simulink model "test"  (R2020b)
settings: Solver=FixedStepAuto  StartTime=0.0  StopTime=10.0  RelTol=1e-3
settings Model: Creator=horse  LastModifiedBy=faith
settings OptimizationCC: BlockReduction=off  ConditionallyExecuteInputs=off  DefaultParameterBehavior=Inlined  OptimizeBlockIOStorage=off
settings HardwareCC: TargetBitPerPointer=64  TargetBitPerSizeT=64  TargetBitPerPtrDiffT=64  TargetLongLongMode=on  TargetIntDivRoundTo=Zero  TargetEndianess=LittleEndian  TargetWordSize=64  TargetHWDeviceType=Generic->Custom  ProdEqTarget=off
settings RTWCC: Description=SystemVerilog DPI Component Generator  SystemTargetFile=systemverilog_dpi_grt.tlc  TemplateMakefile=systemverilog_dpi_grt_default_tmf
settings CodeAppCC: MaxIdLength=256
settings DPIGRTTargetCC: TargetFcnLib=ansi_tfl_table_tmw.mat  GenFloatMathFcnCalls=NOT IN USE  TargetLangStandard=C89/C90 (ANSI)  CodeReplacementLibrary=None  UtilityFuncGeneration=Auto  MultiwordTypeDef=System defined  MultiwordLength=2048  DynamicStringBufferSize=256  GenerateFullHeader=on  InferredTypesCompatibility=off  GenerateSampleERTMain=off  GenerateTestInterfaces=off  ModelReferenceCompliant=on  ParMdlRefBuildCompliant=on  CompOptLevelCompliant=off  ConcurrentExecutionCompliant=off  IncludeMdlTerminateFcn=on  CombineOutputUpdateFcns=off  CombineSignalStateStructs=on  GroupInternalDataByFunction=off  SuppressErrorStatus=off  IncludeFileDelimiter=Auto  ERTCustomFileBanners=off  SupportAbsoluteTime=on  LogVarNameModifier=rt_  MatFileLogging=off  CodeInterfacePackaging=Reusable function  PurelyIntegerCode=off  SupportNonFinite=on  SupportComplex=on  SupportContinuousTime=on  SupportNonInlinedSFcns=on  RemoveDisableFunc=off  RemoveResetFunc=off  SupportVariableSizeSignals=off  ParenthesesLevel=Nominal  CastingMode=Nominal  MATLABClassNameForMDSCustomization=Simulink.SoftwareTarget.TargetSpecificTriggerConfigurationBase  ModelStepFunctionPrototypeControlCompliant=off  CPPClassGenCompliant=off  AutosarCompliant=off  MDXCompliant=off  GRTInterface=off  GenerateAllocFcn=on  UseToolchainInfoCompliant=on  GenerateSharedConstants=on  CoderGroups=[]  AccessMethods=[]  LookupTableObjectStructAxisOrder=1,2,3,4,...  LUTObjectStructOrderExplicitValues=Size,Breakpoints,Table  LUTObjectStructOrderEvenSpacing=Size,Breakpoints,Table  ArrayLayout=Column-major  UnsupportedSFcnMsg=error  ERTHeaderFileRootName=$R$E  ERTSourceFileRootName=$R$E  ERTDataFileRootName=$R_data  RTWCAPISignals=on  RTWCAPIParams=off  RTWCAPIStates=off  RTWCAPIRootIO=off  ExtMode=off  ExtModeTransport=0  ExtModeStaticAlloc=off  ExtModeStaticAllocSize=1000000  ExtModeTesting=off  ExtModeMexFile=ext_comm  GenerateASAP2=off  MultiInstanceErrorCode=Error  DPICustomizeSystemVerilogCode=off  DPISystemVerilogTemplate=svdpi_event.vgt  DPIReportRunTimeError=off  DPIRunTimeErrorSeverity=Fatal  DPIGenerateTestBench=off  DPITestBenchSimulator=Mentor Graphics Questasim  DPITestPointAccessFcnInterface=None  DPIFixedPointDataType=CompatibleCType  DPIPortConnection=Port list  DPICompositeDataType=Flattened

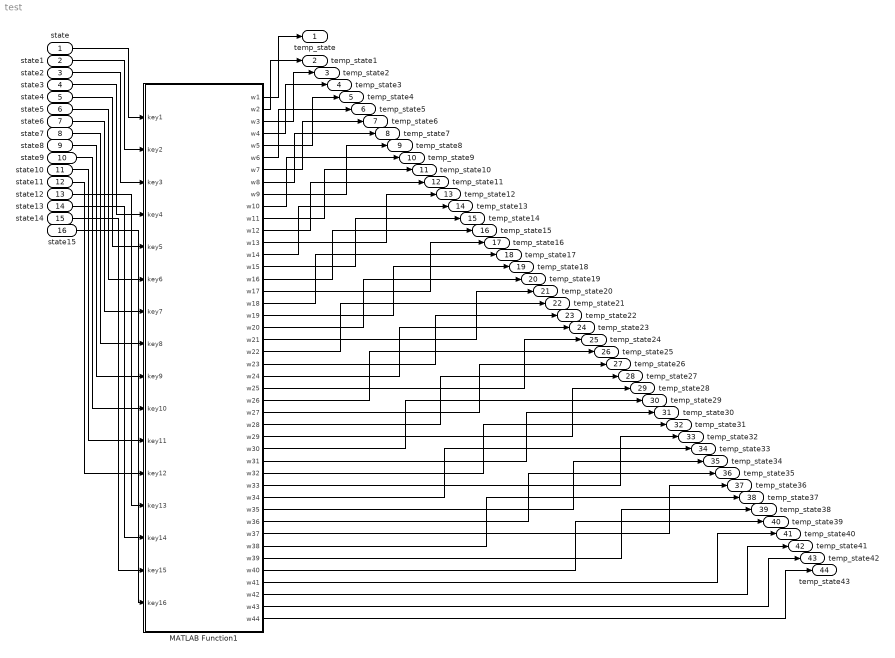
== system test ==
  state : Inport  OutDataTypeStr=uint8
  state1 : Inport  Port=2  OutDataTypeStr=uint8
  state2 : Inport  Port=3  OutDataTypeStr=uint8
  state3 : Inport  Port=4  OutDataTypeStr=uint8
  state4 : Inport  Port=5  OutDataTypeStr=uint8
  state5 : Inport  Port=6  OutDataTypeStr=uint8
  state6 : Inport  Port=7  OutDataTypeStr=uint8
  state7 : Inport  Port=8  OutDataTypeStr=uint8
  state8 : Inport  Port=9  OutDataTypeStr=uint8
  state9 : Inport  Port=10  OutDataTypeStr=uint8
  state10 : Inport  Port=11  OutDataTypeStr=uint8
  state11 : Inport  Port=12  OutDataTypeStr=uint8
  state12 : Inport  Port=13  OutDataTypeStr=uint8
  state13 : Inport  Port=14  OutDataTypeStr=uint8
  state14 : Inport  Port=15  OutDataTypeStr=uint8
  state15 : Inport  Port=16  OutDataTypeStr=uint8
  MATLAB Function1 : MATLAB Function  TreatAsAtomicUnit=on
  temp_state : Outport  OutDataTypeStr=uint32  VectorParamsAs1DForOutWhenUnconnected=off
  temp_state1 : Outport  Port=2  OutDataTypeStr=uint32  VectorParamsAs1DForOutWhenUnconnected=off
  temp_state2 : Outport  Port=3  OutDataTypeStr=uint32  VectorParamsAs1DForOutWhenUnconnected=off
  temp_state3 : Outport  Port=4  OutDataTypeStr=uint32  VectorParamsAs1DForOutWhenUnconnected=off
  temp_state4 : Outport  Port=5  OutDataTypeStr=uint32  VectorParamsAs1DForOutWhenUnconnected=off
  temp_state5 : Outport  Port=6  OutDataTypeStr=uint32  VectorParamsAs1DForOutWhenUnconnected=off
  temp_state6 : Outport  Port=7  OutDataTypeStr=uint32  VectorParamsAs1DForOutWhenUnconnected=off
  temp_state7 : Outport  Port=8  OutDataTypeStr=uint32  VectorParamsAs1DForOutWhenUnconnected=off
  temp_state8 : Outport  Port=9  OutDataTypeStr=uint32  VectorParamsAs1DForOutWhenUnconnected=off
  temp_state9 : Outport  Port=10  OutDataTypeStr=uint32  VectorParamsAs1DForOutWhenUnconnected=off
  temp_state10 : Outport  Port=11  OutDataTypeStr=uint32  VectorParamsAs1DForOutWhenUnconnected=off
  temp_state11 : Outport  Port=12  OutDataTypeStr=uint32  VectorParamsAs1DForOutWhenUnconnected=off
  temp_state12 : Outport  Port=13  OutDataTypeStr=uint32  VectorParamsAs1DForOutWhenUnconnected=off
  temp_state13 : Outport  Port=14  OutDataTypeStr=uint32  VectorParamsAs1DForOutWhenUnconnected=off
  temp_state14 : Outport  Port=15  OutDataTypeStr=uint32  VectorParamsAs1DForOutWhenUnconnected=off
  temp_state15 : Outport  Port=16  OutDataTypeStr=uint32  VectorParamsAs1DForOutWhenUnconnected=off
  temp_state16 : Outport  Port=17  OutDataTypeStr=uint32  VectorParamsAs1DForOutWhenUnconnected=off
  temp_state17 : Outport  Port=18  OutDataTypeStr=uint32  VectorParamsAs1DForOutWhenUnconnected=off
  temp_state18 : Outport  Port=19  OutDataTypeStr=uint32  VectorParamsAs1DForOutWhenUnconnected=off
  temp_state19 : Outport  Port=20  OutDataTypeStr=uint32  VectorParamsAs1DForOutWhenUnconnected=off
  temp_state20 : Outport  Port=21  OutDataTypeStr=uint32  VectorParamsAs1DForOutWhenUnconnected=off
  temp_state21 : Outport  Port=22  OutDataTypeStr=uint32  VectorParamsAs1DForOutWhenUnconnected=off
  temp_state22 : Outport  Port=23  OutDataTypeStr=uint32  VectorParamsAs1DForOutWhenUnconnected=off
  temp_state23 : Outport  Port=24  OutDataTypeStr=uint32  VectorParamsAs1DForOutWhenUnconnected=off
  temp_state24 : Outport  Port=25  OutDataTypeStr=uint32  VectorParamsAs1DForOutWhenUnconnected=off
  temp_state25 : Outport  Port=26  OutDataTypeStr=uint32  VectorParamsAs1DForOutWhenUnconnected=off
  temp_state26 : Outport  Port=27  OutDataTypeStr=uint32  VectorParamsAs1DForOutWhenUnconnected=off
  temp_state27 : Outport  Port=28  OutDataTypeStr=uint32  VectorParamsAs1DForOutWhenUnconnected=off
  temp_state28 : Outport  Port=29  OutDataTypeStr=uint32  VectorParamsAs1DForOutWhenUnconnected=off
  temp_state29 : Outport  Port=30  OutDataTypeStr=uint32  VectorParamsAs1DForOutWhenUnconnected=off
  temp_state30 : Outport  Port=31  OutDataTypeStr=uint32  VectorParamsAs1DForOutWhenUnconnected=off
  temp_state31 : Outport  Port=32  OutDataTypeStr=uint32  VectorParamsAs1DForOutWhenUnconnected=off
  temp_state32 : Outport  Port=33  OutDataTypeStr=uint32  VectorParamsAs1DForOutWhenUnconnected=off
  temp_state33 : Outport  Port=34  OutDataTypeStr=uint32  VectorParamsAs1DForOutWhenUnconnected=off
  temp_state34 : Outport  Port=35  OutDataTypeStr=uint32  VectorParamsAs1DForOutWhenUnconnected=off
  temp_state35 : Outport  Port=36  OutDataTypeStr=uint32  VectorParamsAs1DForOutWhenUnconnected=off
  temp_state36 : Outport  Port=37  OutDataTypeStr=uint32  VectorParamsAs1DForOutWhenUnconnected=off
  temp_state37 : Outport  Port=38  OutDataTypeStr=uint32  VectorParamsAs1DForOutWhenUnconnected=off
  temp_state38 : Outport  Port=39  OutDataTypeStr=uint32  VectorParamsAs1DForOutWhenUnconnected=off
  temp_state39 : Outport  Port=40  OutDataTypeStr=uint32  VectorParamsAs1DForOutWhenUnconnected=off
  temp_state40 : Outport  Port=41  OutDataTypeStr=uint32  VectorParamsAs1DForOutWhenUnconnected=off
  temp_state41 : Outport  Port=42  OutDataTypeStr=uint32  VectorParamsAs1DForOutWhenUnconnected=off
  temp_state42 : Outport  Port=43  OutDataTypeStr=uint32  VectorParamsAs1DForOutWhenUnconnected=off
  temp_state43 : Outport  Port=44  OutDataTypeStr=uint32  VectorParamsAs1DForOutWhenUnconnected=off
  wires:
  state/1 -> MATLAB Function1/1(key1)
  state1/1 -> MATLAB Function1/2(key2)
  state2/1 -> MATLAB Function1/3(key3)
  state3/1 -> MATLAB Function1/4(key4)
  state4/1 -> MATLAB Function1/5(key5)
  state5/1 -> MATLAB Function1/6(key6)
  state6/1 -> MATLAB Function1/7(key7)
  state7/1 -> MATLAB Function1/8(key8)
  state8/1 -> MATLAB Function1/9(key9)
  state9/1 -> MATLAB Function1/10(key10)
  state11/1 -> MATLAB Function1/12(key12)
  state10/1 -> MATLAB Function1/11(key11)
  state12/1 -> MATLAB Function1/13(key13)
  state13/1 -> MATLAB Function1/14(key14)
  state14/1 -> MATLAB Function1/15(key15)
  state15/1 -> MATLAB Function1/16(key16)
  MATLAB Function1/1(w1) -> temp_state/1
  MATLAB Function1/2(w2) -> temp_state1/1
  MATLAB Function1/3(w3) -> temp_state2/1
  MATLAB Function1/4(w4) -> temp_state3/1
  MATLAB Function1/5(w5) -> temp_state4/1
  MATLAB Function1/6(w6) -> temp_state5/1
  MATLAB Function1/7(w7) -> temp_state6/1
  MATLAB Function1/8(w8) -> temp_state7/1
  MATLAB Function1/9(w9) -> temp_state8/1
  MATLAB Function1/10(w10) -> temp_state9/1
  MATLAB Function1/11(w11) -> temp_state10/1
  MATLAB Function1/12(w12) -> temp_state11/1
  MATLAB Function1/13(w13) -> temp_state12/1
  MATLAB Function1/14(w14) -> temp_state13/1
  MATLAB Function1/15(w15) -> temp_state14/1
  MATLAB Function1/16(w16) -> temp_state15/1
  MATLAB Function1/17(w17) -> temp_state16/1
  MATLAB Function1/18(w18) -> temp_state17/1
  MATLAB Function1/19(w19) -> temp_state18/1
  MATLAB Function1/20(w20) -> temp_state19/1
  MATLAB Function1/21(w21) -> temp_state20/1
  MATLAB Function1/22(w22) -> temp_state21/1
  MATLAB Function1/23(w23) -> temp_state22/1
  MATLAB Function1/24(w24) -> temp_state23/1
  MATLAB Function1/25(w25) -> temp_state24/1
  MATLAB Function1/26(w26) -> temp_state25/1
  MATLAB Function1/27(w27) -> temp_state26/1
  MATLAB Function1/28(w28) -> temp_state27/1
  MATLAB Function1/29(w29) -> temp_state28/1
  MATLAB Function1/30(w30) -> temp_state29/1
  MATLAB Function1/31(w31) -> temp_state30/1
  MATLAB Function1/32(w32) -> temp_state31/1
  MATLAB Function1/33(w33) -> temp_state32/1
  MATLAB Function1/34(w34) -> temp_state33/1
  MATLAB Function1/35(w35) -> temp_state34/1
  MATLAB Function1/36(w36) -> temp_state35/1
  MATLAB Function1/37(w37) -> temp_state36/1
  MATLAB Function1/38(w38) -> temp_state37/1
  MATLAB Function1/39(w39) -> temp_state38/1
  MATLAB Function1/40(w40) -> temp_state39/1
  MATLAB Function1/41(w41) -> temp_state40/1
  MATLAB Function1/42(w42) -> temp_state41/1
  MATLAB Function1/43(w43) -> temp_state42/1
  MATLAB Function1/44(w44) -> temp_state43/1

== matlab function test/MATLAB Function1 ==
  data: key1 input; w1 output; key2 input; key3 input; key4 input; key5 input; key6 input; key7 input; key8 input; key9 input; key10 input; key11 input; key12 input; key13 input; key14 input; key15 input; key16 input; w2 output; w3 output; w4 output; w5 output; w6 output; w7 output; w8 output; w9 output; w10 output; w11 output; w12 output; w13 output; w14 output; w15 output; w16 output; w17 output; w18 output; w19 output; w20 output; w21 output; w22 output; w23 output; w24 output; w25 output; w26 output; w27 output; w28 output; w29 output; w30 output; w31 output; w32 output; w33 output; w34 output; w35 output; w36 output; w37 output; w38 output; w39 output; w40 output; w41 output; w42 output; w43 output; w44 output
function [w1, w2, w3, w4, w5, w6, w7, w8, w9, w10, w11, w12, w13, w14, w15, w16, w17, w18, w19, w20, w21, w22, w23, w24, w25, w26, w27, w28, w29, w30, w31, w32, w33, w34, w35, w36, w37, w38, w39, w40, w41, w42, w43, w44] = KeyExpansion(key1, key2, key3, key4, key5, key6, key7, key8, key9, key10, key11, key12, key13, key14, key15, key16)

%     round constant do not delete
    Rcon = uint32([0x8d000000 0x01000000 0x02000000 0x04000000 0x08000000 0x10000000 0x20000000 0x40000000 0x80000000 0x1b000000 0x36000000 ]);
    
    w = uint32(zeros(1,44));
	temp = uint32(0);
	i = uint8(1);

    % first loop worked out:

    % iteration 1:
    w(1) = w(1) + uint32(key1);
    w(1) = bitsll(w(1), 8);
    w(1) = w(1) + uint32(key2);
    w(1) = bitsll(w(1), 8);
    w(1) = w(1) + uint32(key3);
    w(1) = bitsll(w(1), 8);
    w(1) = w(1) + uint32(key4);

    % iteration 2:
    w(2) = w(2) + uint32(key5);
    w(2) = bitsll(w(2), 8);
    w(2) = w(2) + uint32(key6);
    w(2) = bitsll(w(2), 8);
    w(2) = w(2) + uint32(key7);
    w(2) = bitsll(w(2), 8);
    w(2) = w(2) + uint32(key8);

    % iteration 3:
    w(3) = w(3) + uint32(key9);
    w(3) = bitsll(w(3), 8);
    w(3) = w(3) + uint32(key10);
    w(3) = bitsll(w(3), 8);
    w(3) = w(3) + uint32(key11);
    w(3) = bitsll(w(3), 8);
    w(3) = w(3) + uint32(key12);

    % iteration 4:
    w(4) = w(4) + uint32(key13);
    w(4) = bitsll(w(4), 8);
    w(4) = w(4) + uint32(key14);
    w(4) = bitsll(w(4), 8);
    w(4) = w(4) + uint32(key15);
    w(4) = bitsll(w(4), 8);
    w(4) = w(4) + uint32(key16);

%     %the rest of the blocks
%     for i = 4:43
% 		temp = uint32(w(i));
%         if (mod(i, 4) == 0) % this has been changed 
% 			temp = uint32(RotWord(temp));
% 			temp = uint32(SubWord(temp));
% 			temp = uint32(bitxor(temp, Rcon(floor((i+1) / 4 )+1))); % might need to be i + 1
%         end
% 		w(i+1) = bitxor(w(i - 3), temp);
%     end
	
    w1 = w(1);
    w2 = w(2);
    w3 = w(3);
    w4 = w(4); 
    
    w5_temp = w(4);
    w5 = uint32(RotWord(w5_temp));
    w5 = uint32(SubWord(w5_temp));
    w5 = uint32(bitxor(w5_temp, Rcon(2))); 
    w5 = bitxor(w1, w5_temp);
    
    w6 = bitxor(w5, w2);
    w7 = bitxor(w6, w3);
    w8 = bitxor(w7, w4);

    w9_temp = w(8);
    w9 = uint32(RotWord(w9_temp));
    w9 = uint32(SubWord(w9_temp));
    w9 = uint32(bitxor(w9_temp, Rcon(3))); 
    w9 = bitxor(w5, w9_temp);
     
    w10 = bitxor(w9, w6);
    w11 = bitxor(w10, w7);
    w12 = bitxor(w11, w8);
    
    w13_temp = w(12);
    w13 = uint32(RotWord(w13_temp));
    w13 = uint32(SubWord(w13_temp));
    w13 = uint32(bitxor(w13_temp, Rcon(4))); 
    w13 = bitxor(w9, w13_temp);

    w14 = w(14);
    w15 = w(15);
    w16 = w(16);
    
    w17_temp = w(16);
    w17 = uint32(RotWord(w17_temp));
    w17 = uint32(SubWord(w17_temp));
    w17 = uint32(bitxor(w17_temp, Rcon(5))); 
    w17 = bitxor(w13, w17_temp);
    
    w18 = bitxor(w17, w14);
    w19 = bitxor(w18, w15);
    w20 = bitxor(w19, w16);
    
    w21_temp = w(20);
    w21 = uint32(RotWord(w21_temp));
    w21 = uint32(SubWord(w21_temp));
    w21 = uint32(bitxor(w21_temp, Rcon(6))); 
    w21 = bitxor(w17, w21_temp);
    
    w22 = bitxor(w21, w18);
    w23 = bitxor(w22, w19);
    w24 = bitxor(w23, w20);
    
    w25_temp = w(24);
    w25 = uint32(RotWord(w25_temp));
    w25 = uint32(SubWord(w25_temp));
    w25 = uint32(bitxor(w25_temp, Rcon(7))); 
    w25 = bitxor(w21, w25_temp);
    
    w26 = bitxor(w24, w21);
    w27 = bitxor(w25, w22);
    w28 = bitxor(w26, w23);
   
    w29_temp = w(28);
    w29 = uint32(RotWord(w29_temp));
    w29 = uint32(SubWord(w29_temp));
    w29 = uint32(bitxor(w29_temp, Rcon(8))); 
    w29 = bitxor(w25, w29_temp);
   
    w30 = bitxor(w29, w26);
    w31 = bitxor(w30, w27);
    w32 = bitxor(w31, w28);
   
    w33_temp = w(32);
    w33 = uint32(RotWord(w33_temp));
    w33 = uint32(SubWord(w33_temp));
    w33 = uint32(bitxor(w33_temp, Rcon(9))); 
    w33 = bitxor(w29, w33_temp);
   
    w34 = bitxor(w33, w30);
    w35 = bitxor(w34, w31);
    w36 = bitxor(w35, w32);
   
    w37_temp = w(36);
    w37 = uint32(RotWord(w37_temp));
    w37 = uint32(SubWord(w37_temp));
    w37 = uint32(bitxor(w37_temp, Rcon(10))); 
    w37 = bitxor(w33, w37_temp);
   
    w38 = bitxor(w37, w34);
    w39 = bitxor(w38, w35);
    w40 = bitxor(w39, w36);
   
    w41_temp = w(40);
    w41 = uint32(RotWord(w41_temp));
    w41 = uint32(SubWord(w41_temp));
    w41 = uint32(bitxor(w41_temp, Rcon(11))); 
    w41 = bitxor(w37, w41_temp);
   
    w42 = bitxor(w41, w38);
    w43 = bitxor(w42, w39);
    w44 = bitxor(w43, w40);
end
